simulink model "simulink_ompc_discrete"  (R2022b)
settings: Solver=ode8  StartTime=0.0  StopTime=time  FixedStep=Ts  RelTol=1e-3
values from neighbouring files (symbols this model uses):
  A_bar = [Ad, Z_unknown; zeros(n_disturbances, n_states), zeros(n_disturbances)]    [plik_generujDane.m]
  B_bar = [Bd; zeros(n_disturbances, size(Bd, 2))]    [plik_generujDane.m]
  Bd = Bd(:, 1:size(B, 2))    [plik_generujDane.m]
  C_bar = [C_measured, zeros(size(C_measured, 1), n_disturbances)]    [plik_generujDane.m]
  C_measured = [C_measured zeros(size(C_measured,1),1)]    [plik_generujDane.m]
  D = Dm    [generateBuilding.m]    (also in generateFloor.m; generateRoom.m = 0; heatPump.m = 0; mergePumpBuilding.m)
  K = P_pred * C' / (C * P_pred * C' + R)    [KalmanFilter.m]
  Kz = zeros(ny * na, nd * na)    [create_Kz_matrix.m]    (also in ompc_cost.m = [-K,eye(nu),zeros(nu,(nc-1)*nu)]; ompc_cost_tracking.m = [-K,eye(nu),zeros(nu,(nc-1)*nu),[K*Kxr+Kur zeros(nu,nya-nu)]; plik_generujDane.m = create_Kz_matrix(Ad, Cd, Zd, na))
  L = vecNeighbors(1,1)    [genRoomParams.m]    (also in generateParameters.m; generateRoom.m; model_expanded.m = 6; model_parameters.m)
  na = 72    [plik_generujDane.m]
  nc = 48    [plik_generujDane.m]
  npred = 72    [plik_generujDane.m]
  Qflow = table2array(roomEquipment(end,:))    [plik_generujDane.m]
  Sc = Spsi(nx+1:end,nx+1:end)    [ompc_cost.m]    (also in ompc_cost_tracking.m = Spsi(nx+1:nx+nuc,nx+1:nx+nuc))
  Scr = Spsi(nx+1:nx+nuc,nx+nuc+1:end)    [ompc_cost_tracking.m]
  Sxc = Spsi(1:nx,nx+1:end)    [ompc_cost.m]    (also in ompc_cost_tracking.m = Spsi(1:nx,nx+1:nx+nuc))
  time = 3600*24*7    (= 604800)    [plik_generujDane.m]
  trajDist = [d1Temp d2Temp d3Temp d4Temp d5Temp d6Temp d7Temp ... (first row only)    [plik_generujDane.m]
  trajPrice = [trajPrice trajPrice trajPrice trajPrice trajPrice trajPrice trajPrice]    [plik_generujDane.m]
  trajRef = [trajRef trajRef trajRef trajRef trajRef trajRef trajRef]    [plik_generujDane.m]
  Ts = 1200    [plik_generujDane.m]
  umax = [umax; P_MAX]    [plik_generujDane.m]
  umin = [umin; P_MIN]    [plik_generujDane.m]
  w_PumpCost = 1.5    [plik_generujDane.m]
  x0 = x0'    [initialStates.m]    (also in plik_generujDane.m = [x0;T_buf])
  xmax = [xmax [Ta_max xmax0 Twall_max Twall_max Tp_max T_return_max]]    [initialStates.m]    (also in plik_generujDane.m = [xmax; T_bufMAX])
  xmin = [xmin [Ta_min xmin0 Twall_min Twall_min Tp_min T_return_min]]    [initialStates.m]    (also in plik_generujDane.m = [xmin; T_bufMIN])
  ymax = [ymax; T_bufMAX]    [plik_generujDane.m]
  ymin = [ymin; T_bufMIN]    [plik_generujDane.m]
  Z = [Z zeros(nZ, nZmcol-3); Zm(:,1:2) zeros(nZm, nZcol-3) Zm(:,3:end)]    [generateBuilding.m]    (also in generateFloor.m = [Z zeros(nZ,1); Zm(:,1:2) zeros(nZm,nZcol-2) Zm(:,3)]; generateRoom.m = [0 0 0 0 0 0 1/Ca; heatPump.m = [area_buf*U -m_dot.*cw m_dot.*cw]/C_bufor; mergeFloorModels.m = Z0)
  Z_bar_known = [Z_known; zeros(n_disturbances, size(Z_known, 2))]    [plik_generujDane.m]
  Zd = Bd(:, size(B,2)+1:end)    [plik_generujDane.m]
  zoneWaterIndex = [zoneWaterIndex size(A,1)-1]    [plik_generujDane.m]
undefined symbols (not defined in the file or in its folder): Ad, Cd, priceCost
settings Model: Creator=artur  LastModifiedBy=artur

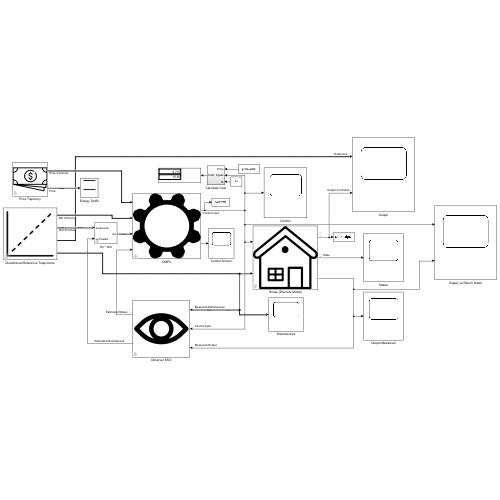
[thumbnail: Simulink's stored preview of the top-level diagram]
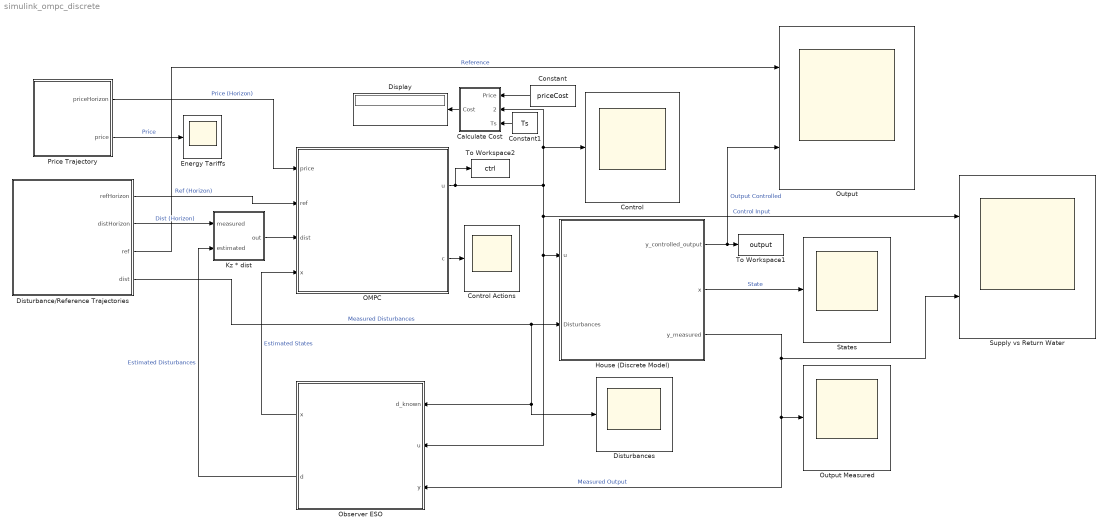
== system simulink_ompc_discrete ==
  Calculate Cost : Subsystem
  Constant : Constant  Value=priceCost
  Constant1 : Constant  Value=Ts
  Control : Scope
  Control Actions : Scope
  Display : Display
  Disturbance/Reference Trajectories : Subsystem  mask{time=time, Ts=Ts, na=na, refValues=trajRef, distValues=trajDist}
      mask prompts: time "Czas symulacji"; Ts "Okres próbkowania"; na "Horyzont trajektorii"; refValues "Trajektoria referencyjna"; distValues "Trajektoria zakłóceń"
      mask Display: image('C:\Users\artur\OneDrive\Dokumenty\MATLAB\Magisterka\model\images\plot-icon.svg'); % Use "Edit Image" on toolstrip to change.
  Disturbances : Scope
  Energy Tariffs : Scope
  House (Discrete Model) : Subsystem  mask{A=Ad, B=Bd, C=Cd, C_measured=C_measured, D=D, Z=Zd, x0=x0}
      mask prompts: A "Macierz A:"; B "Macierz B"; C "Macierz C sterowane"; C_measured "Macierz C mierzone"; D "Macierz D"; Z "Macierz zakłóceń Z"; x0 "War. początkowe"
      mask DialogControl ParameterGroupVar Prompt: Parametry modelu
      mask Display: image('C:\Users\artur\OneDrive\Dokumenty\MATLAB\Magisterka\model\images\house-icon.svg'); % Use "Edit Image" on toolstrip to change.
  Kz * dist : Subsystem  mask{Kz=Kz, na=na}
  OMPC : Subsystem  mask{A=Ad, B=Bd, C=Cd, nc=nc, npred=npred, na=na, w=w_PumpCost, Sxc=Sxc, Scr=Scr, Sc=Sc, K=K, umax=umax, umin=umin, ymax=ymax, ymin=ymin, xmax=xmax, xmin=xmin, M=zoneWaterIndex, Qflow=Qflow}
      mask prompts: A "Macierz A"; B "Macierz  B"; C "Macierz C"; nc "Liczba zmiennych decyzyjnych"; npred "Horyzont predykcji"; na "Horyzont trajektorii"; w "Waga kosztów cen energii"; Sxc "Macierz Sxc"; Scr "Macierz Scr"; Sc "Macierz Sc"; K "Macierz K"; M "Wektor indeksów stanów wody w strefie"; Qflow "PPrzepływy w pętlach grzewczych"
      mask DialogControl ParameterGroupVar Prompt: Parametry modelu
      mask DialogControl Container3 Prompt: Parametry regulatora
      mask DialogControl Container4 Prompt: Ograniczenia
      mask Display: image('C:\Users\artur\OneDrive\Dokumenty\MATLAB\Magisterka\model\images\cogwheel-icon.svg'); % Use "Edit Image" on toolstrip to change.
  Observer ESO : Subsystem  mask{A_bar=A_bar, B_bar=B_bar, C_bar=C_bar, A=Ad, L=L, Z_bar_known=Z_bar_known}
      mask DialogControl Observer Prompt: Parametry Obserwatora
      mask Display: image('C:\Users\artur\OneDrive\Dokumenty\MATLAB\Magisterka\model\images\eye-icon.svg'); % Use "Edit Image" on toolstrip to change.
  Output : Scope  NumInputPorts=2
  Output Measured : Scope
  Price Trajectory : Subsystem  mask{time=time, Ts=Ts, N=nc, refValues=trajPrice}
      mask prompts: time "Czas symulacji"; Ts "Okres próbkowania"; N "Horyzont"; refValues "Trajektoria zmian cen"
      mask Display: image('C:\Users\artur\OneDrive\Dokumenty\MATLAB\Magisterka\model\images\cash-icon.svg'); % Use "Edit Image" on toolstrip to change.
  States : Scope
  Supply vs Return Water : Scope  NumInputPorts=2
  To Workspace1 : ToWorkspace  VariableName=output  SampleTime=-1
      settings: Save2DSignal=2-D array (concatenate along first dimension)
  To Workspace2 : ToWorkspace  VariableName=ctrl  SampleTime=-1
      settings: Save2DSignal=2-D array (concatenate along first dimension)
  wires:
  OMPC/1(u) -> To Workspace2/1, Control/1, Calculate Cost/2(Inputs), Supply vs Return Water/1, House (Discrete Model)/1(u), Observer ESO/2(u)  "Control Input"
  House (Discrete Model)/2(x) -> States/1  "State"
  Disturbance/Reference Trajectories/3(ref) -> Output/1  "Reference"
  Disturbance/Reference Trajectories/1(refHorizon) -> OMPC/2(ref)  "Ref (Horizon)"
  House (Discrete Model)/3(y_measured) -> Supply vs Return Water/2, Output Measured/1, Observer ESO/3(y)  "Measured Output"
  Observer ESO/2(d) -> Kz * dist/2(estimated)  "Estimated Disturbances"
  House (Discrete Model)/1(y_controlled_output) -> Output/2, To Workspace1/1  "Output Controlled"
  Kz * dist/1(out) -> OMPC/3(dist)
  Disturbance/Reference Trajectories/2(distHorizon) -> Kz * dist/1(measured)  "Dist (Horizon)"
  OMPC/2(c) -> Control Actions/1
  Disturbance/Reference Trajectories/4(dist) -> Disturbances/1, Observer ESO/1(d_known), House (Discrete Model)/2(Disturbances)  "Measured Disturbances"
  Price Trajectory/1(priceHorizon) -> OMPC/1(price)  "Price (Horizon)"
  Price Trajectory/2(price) -> Energy Tariffs/1  "Price"
  Calculate Cost/1(Cost) -> Display/1
  Constant/1 -> Calculate Cost/1(Price)
  Constant1/1 -> Calculate Cost/3(Ts)
  Observer ESO/1(x) -> OMPC/4(x)  "Estimated States"

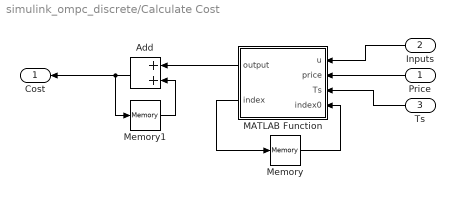
== system simulink_ompc_discrete/Calculate Cost ==
  Price : Inport
  Inputs : Inport  Port=2
  Ts : Inport  Port=3
  Add : Sum
  MATLAB Function : MATLAB Function  TreatAsAtomicUnit=on
  Memory : Memory  InitialCondition=1
  Memory1 : Memory  InitialCondition=[0 0]
  Cost : Outport
  wires:
  Inputs/1 -> MATLAB Function/1(u)
  Price/1 -> MATLAB Function/2(price)
  MATLAB Function/2(index) -> Memory/1
  Memory/1 -> MATLAB Function/4(index0)
  Memory1/1 -> Add/2
  Add/1 -> Cost/1, Memory1/1
  MATLAB Function/1(output) -> Add/1
  Ts/1 -> MATLAB Function/3(Ts)

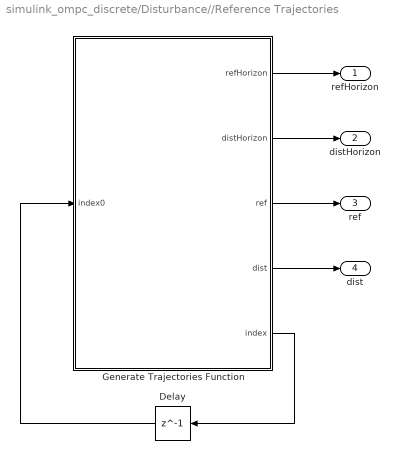
== system simulink_ompc_discrete/Disturbance//Reference Trajectories ==
  Delay : Delay  DelayLength=1  InitialCondition=1
  Generate Trajectories Function : MATLAB Function  TreatAsAtomicUnit=on
  refHorizon : Outport
  distHorizon : Outport  Port=2
  ref : Outport  Port=3
  dist : Outport  Port=4
  wires:
  Generate Trajectories Function/2(distHorizon) -> distHorizon/1
  Generate Trajectories Function/3(ref) -> ref/1
  Generate Trajectories Function/1(refHorizon) -> refHorizon/1
  Generate Trajectories Function/5(index) -> Delay/1
  Delay/1 -> Generate Trajectories Function/1(index0)
  Generate Trajectories Function/4(dist) -> dist/1

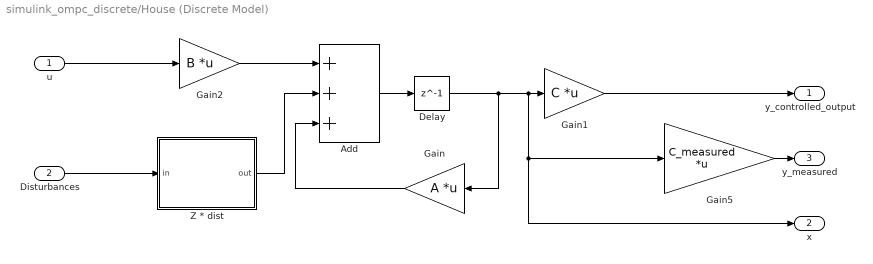
== system simulink_ompc_discrete/House (Discrete Model) ==
  u : Inport
  Disturbances : Inport  Port=2
  Add : Sum  Inputs=+++
  Delay : Delay  DelayLength=1  InitialCondition=x0
  Gain : Gain  Gain=A  Multiplication=Matrix(K*u) (u vector)
  Gain1 : Gain  Gain=C  Multiplication=Matrix(K*u) (u vector)
  Gain2 : Gain  Gain=B  Multiplication=Matrix(K*u) (u vector)
  Gain5 : Gain  Gain=C_measured  Multiplication=Matrix(K*u) (u vector)
  Z * dist : Subsystem  mask{Z=Z}
  y_controlled_output : Outport
  x : Outport  Port=2
  y_measured : Outport  Port=3
  wires:
  u/1 -> Gain2/1
  Delay/1 -> Gain5/1, x/1, Gain1/1, Gain/1
  Add/1 -> Delay/1
  Gain2/1 -> Add/1
  Gain1/1 -> y_controlled_output/1
  Gain/1 -> Add/3
  Disturbances/1 -> Z * dist/1(in)
  Z * dist/1(out) -> Add/2
  Gain5/1 -> y_measured/1

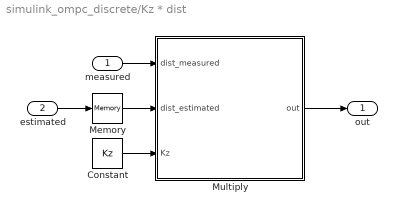
== system simulink_ompc_discrete/Kz * dist ==
  measured : Inport
  estimated : Inport  Port=2
  Constant : Constant  Value=Kz
  Memory : Memory  InitialCondition=zeros(size(Z,2)-6,1)
  Multiply : MATLAB Function  TreatAsAtomicUnit=on
  out : Outport
  wires:
  Multiply/1(out) -> out/1
  measured/1 -> Multiply/1(dist_measured)
  estimated/1 -> Memory/1
  Memory/1 -> Multiply/2(dist_estimated)
  Constant/1 -> Multiply/3(Kz)

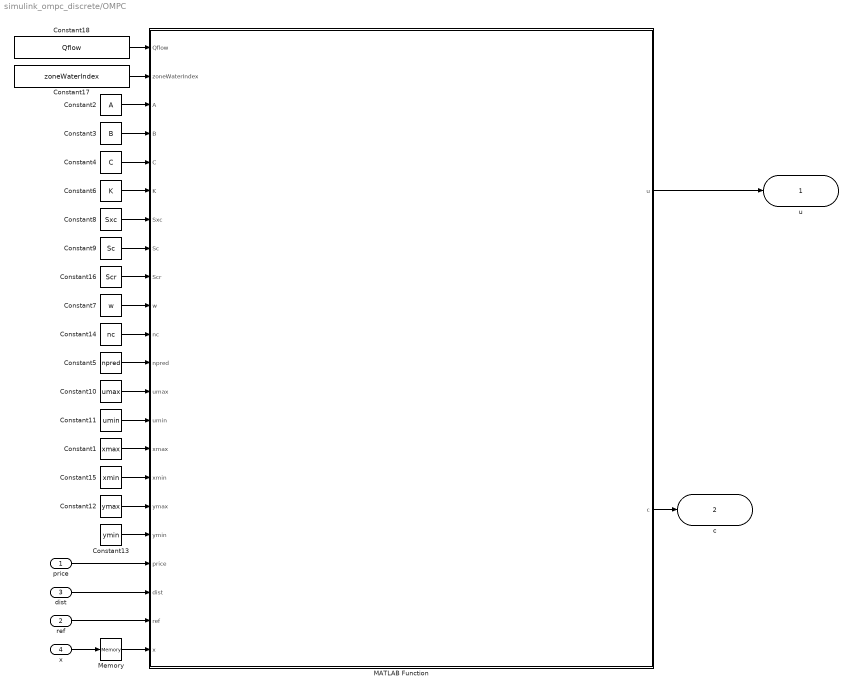
== system simulink_ompc_discrete/OMPC ==
  price : Inport
  ref : Inport  Port=2
  dist : Inport  Port=3
  x : Inport  Port=4
  Constant1 : Constant  Value=xmax  VectorParams1D=off
  Constant10 : Constant  Value=umax  VectorParams1D=off
  Constant11 : Constant  Value=umin  VectorParams1D=off
  Constant12 : Constant  Value=ymax
  Constant13 : Constant  Value=ymin
  Constant14 : Constant  Value=nc
  Constant15 : Constant  Value=xmin
  Constant16 : Constant  Value=Scr  VectorParams1D=off
  Constant17 : Constant  Value=zoneWaterIndex
  Constant18 : Constant  Value=Qflow
  Constant2 : Constant  Value=A
  Constant3 : Constant  Value=B  VectorParams1D=off
  Constant4 : Constant  Value=C  VectorParams1D=off
  Constant5 : Constant  Value=npred
  Constant6 : Constant  Value=K  VectorParams1D=off
  Constant7 : Constant  Value=w
  Constant8 : Constant  Value=Sxc  VectorParams1D=off
  Constant9 : Constant  Value=Sc  VectorParams1D=off
  MATLAB Function : MATLAB Function  TreatAsAtomicUnit=on
  Memory : Memory  InitialCondition=x0
  u : Outport
  c : Outport  Port=2
  wires:
  Constant6/1 -> MATLAB Function/6(K)
  Constant9/1 -> MATLAB Function/8(Sc)
  Constant8/1 -> MATLAB Function/7(Sxc)
  Constant2/1 -> MATLAB Function/3(A)
  Constant4/1 -> MATLAB Function/5(C)
  x/1 -> Memory/1
  Constant3/1 -> MATLAB Function/4(B)
  ref/1 -> MATLAB Function/21(ref)
  Constant10/1 -> MATLAB Function/13(umax)
  Constant11/1 -> MATLAB Function/14(umin)
  Constant12/1 -> MATLAB Function/17(ymax)
  Constant13/1 -> MATLAB Function/18(ymin)
  Memory/1 -> MATLAB Function/22(x)
  MATLAB Function/2(c) -> c/1
  Constant5/1 -> MATLAB Function/12(npred)
  Constant14/1 -> MATLAB Function/11(nc)
  dist/1 -> MATLAB Function/20(dist)
  Constant15/1 -> MATLAB Function/16(xmin)
  Constant1/1 -> MATLAB Function/15(xmax)
  Constant16/1 -> MATLAB Function/9(Scr)
  price/1 -> MATLAB Function/19(price)
  Constant7/1 -> MATLAB Function/10(w)
  Constant17/1 -> MATLAB Function/2(zoneWaterIndex)
  Constant18/1 -> MATLAB Function/1(Qflow)
  MATLAB Function/1(u) -> u/1

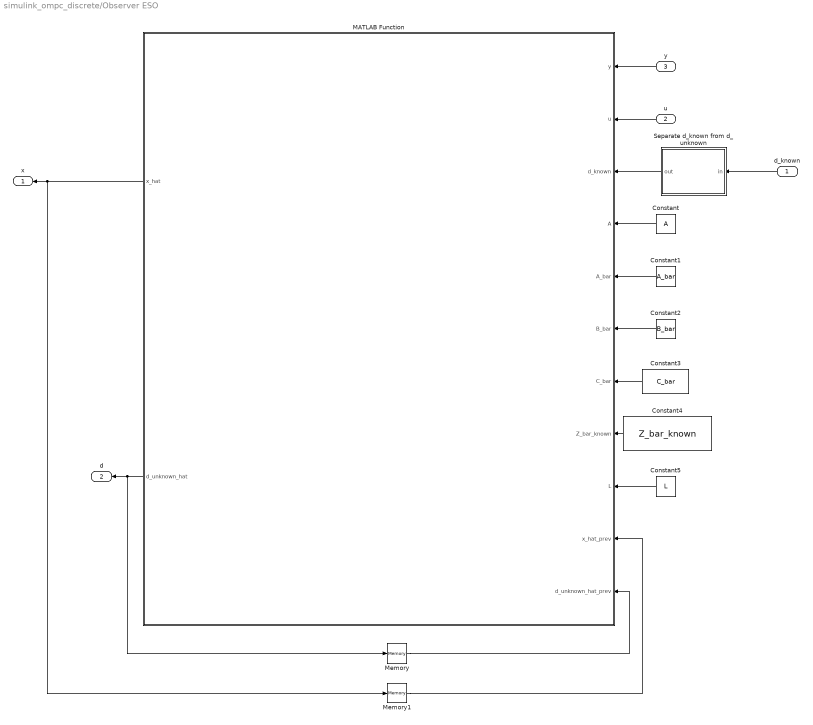
== system simulink_ompc_discrete/Observer ESO ==
  d_known : Inport
  u : Inport  Port=2
  y : Inport  Port=3
  Constant : Constant  Value=A
  Constant1 : Constant  Value=A_bar
  Constant2 : Constant  Value=B_bar
  Constant3 : Constant  Value=C_bar
  Constant4 : Constant  Value=Z_bar_known
  Constant5 : Constant  Value=L
  MATLAB Function : MATLAB Function  TreatAsAtomicUnit=on
  Memory : Memory  InitialCondition=zeros(size(Z,2) - size(Z_bar_known,2),1)
  Memory1 : Memory  InitialCondition=x0
  Separate d_known from d_unknown : MATLAB Function  TreatAsAtomicUnit=on
  x : Outport
  d : Outport  Port=2
  wires:
  MATLAB Function/2(d_unknown_hat) -> Memory/1, d/1
  Memory/1 -> MATLAB Function/11(d_unknown_hat_prev)
  Memory1/1 -> MATLAB Function/10(x_hat_prev)
  MATLAB Function/1(x_hat) -> Memory1/1, x/1
  y/1 -> MATLAB Function/1(y)
  u/1 -> MATLAB Function/2(u)
  Constant/1 -> MATLAB Function/4(A)
  Constant1/1 -> MATLAB Function/5(A_bar)
  Constant2/1 -> MATLAB Function/6(B_bar)
  Constant3/1 -> MATLAB Function/7(C_bar)
  Constant4/1 -> MATLAB Function/8(Z_bar_known)
  Constant5/1 -> MATLAB Function/9(L)
  d_known/1 -> Separate d_known from d_unknown/1(in)
  Separate d_known from d_unknown/1(out) -> MATLAB Function/3(d_known)

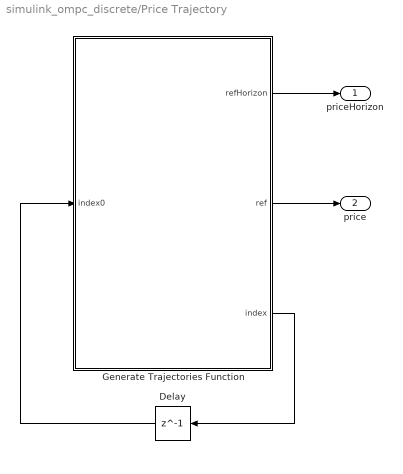
== system simulink_ompc_discrete/Price Trajectory ==
  Delay : Delay  DelayLength=1  InitialCondition=1
  Generate Trajectories Function : MATLAB Function  TreatAsAtomicUnit=on
  priceHorizon : Outport
  price : Outport  Port=2
  wires:
  Generate Trajectories Function/2(ref) -> price/1
  Generate Trajectories Function/1(refHorizon) -> priceHorizon/1
  Generate Trajectories Function/3(index) -> Delay/1
  Delay/1 -> Generate Trajectories Function/1(index0)

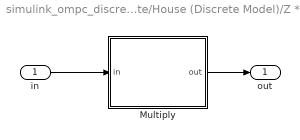
== system simulink_ompc_discrete/House (Discrete Model)/Z * dist ==
  in : Inport
  Multiply : MATLAB Function  TreatAsAtomicUnit=on
  out : Outport
  wires:
  Multiply/1(out) -> out/1
  in/1 -> Multiply/1(in)

== matlab function simulink_ompc_discrete/Observer ESO/MATLAB Function ==
  data: y input; u input; x_hat output; d_unknown_hat output; d_known input; A input; A_bar input; B_bar input; C_bar input; Z_bar_known input; L input; x_hat_prev input; d_unknown_hat_prev input
function [x_hat, d_unknown_hat] = observerESO(y, u, d_known, A, A_bar, B_bar, C_bar, Z_bar_known, L, x_hat_prev, d_unknown_hat_prev)

nx = size(A, 1);

% Rozszerzone stany
x_bar_hat = [x_hat_prev; d_unknown_hat_prev];
y_hat = C_bar * x_bar_hat;

% Aktualizacja estymacji
x_bar_hat = A_bar * x_bar_hat + B_bar * u + Z_bar_known * d_known + L * (y - y_hat);

x_hat = x_bar_hat(1:nx); % Estymowane stany
d_unknown_hat = x_bar_hat(nx+1:end); % Estymowane nieznane zakłócenia
end

== matlab function simulink_ompc_discrete/Observer ESO/Separate d_known from d_unknown ==
  data: in input; out output
function out = fcn(in)

out = in(1:6,:);

== matlab function simulink_ompc_discrete/House (Discrete Model)/Z * dist/Multiply ==
  data: in input; out output; Z parameter
function out = fcn(in, Z)
out = Z*in;

== matlab function simulink_ompc_discrete/Price Trajectory/Generate Trajectories Function ==
  data: refHorizon output size=na*ny; ref output size=ny; time parameter; Ts parameter; N parameter; refValues parameter; index output; index0 input
function [refHorizon,ref,index] = fcn(time, Ts, N, refValues, index0)

flag = 1;
[~, refHorizon, ref] = generateTrajectory(refValues,flag,time,Ts,N,index0);

index = index0 + 1;

== matlab function simulink_ompc_discrete/Calculate Cost/MATLAB Function ==
  data: u input; output output; price input; Ts input; index0 input; index output
function [output, index] = fcn(u, price, Ts, index0)

% u [W]
% price [kWh]

%przekonwertuj na kWh
t_base = Ts/3600;

cost = u(end,end)/1000*t_base * price(index0);
power = u(end,end)/1000*t_base;
output = [cost power];
index = index0 + 1;

== matlab function simulink_ompc_discrete/Disturbance//Reference Trajectories/Generate Trajectories Function ==
  data: refHorizon output size=na*ny; distHorizon output size=na*nz; ref output size=ny; dist output size=nz; time parameter; Ts parameter; na parameter; refValues parameter; distValues parameter; index output; index0 input
function [refHorizon,distHorizon,ref,dist,index] = fcn(time, Ts, na, refValues, distValues, index0)

mode = 1;
[~, refHorizon, ref] = generateTrajectory(refValues,mode,time,Ts,na,index0);

N = size(refValues,1);

for i = 1:N-1
    for j = 1:na-1
        if refHorizon(i + (j-1)*N) > refHorizon(i+j*N)
            refHorizon(i+j*N) = refHorizon(i + (j-1)*N);
        end
    end
end

mode = 2;
[~, distHorizon, dist] = generateTrajectory(distValues,mode,time,Ts,na,index0);

index = index0 + 1;

== matlab function simulink_ompc_discrete/Kz * dist/Multiply ==
  data: dist_measured input; dist_estimated input; out output size=ny*na; Kz input
function out = fcn(dist_measured,dist_estimated, Kz)

%--------------------------------------------------------------------------
%Stwórz wektor sygnałów zakłócających z danych pomiarowych oraz estymacji
len_measured = length(dist_measured);
len_estimated = length(dist_estimated);
len_repeating = 6 + len_estimated; %6 wynika z liczby zakłóceń mierzalnych
N = len_measured / len_repeating;
disturbance_vector = zeros(size(dist_measured));
idx = 1;
for i = 1:N
    start_idx = (i-1) * len_repeating + 1;
    disturbance_vector(idx:idx+2) = dist_measured(start_idx:start_idx+2);
    idx = idx + 6;
    disturbance_vector(idx:idx+len_estimated-1) = dist_estimated;
    idx = idx + len_estimated;
end

out = Kz*disturbance_vector;

== matlab function simulink_ompc_discrete/OMPC/MATLAB Function ==
  data: Qflow input; zoneWaterIndex input; A input; B input; C input; K input; Sxc input; Sc input; Scr input; w input; nc input; npred input; umax input; umin input; xmax input; xmin input; ymax input; ymin input; price input; dist input; ref input; x input; u output; c output
function [u,c] = fcn(Qflow,zoneWaterIndex,A,B,C,K,Sxc,Sc,Scr,w,nc,npred,umax,umin,xmax,xmin,ymax,ymin,price,dist,ref,x)

for i = 1:size(umin,1)-1
    umin(i) = x(zoneWaterIndex(i));
end

[u,ctrl] = ompc_law(A,B,C,K,Sxc,Sc,Scr,Qflow,zoneWaterIndex,umax,umin,xmax,xmin,ymax,ymin,w,nc,npred,price,ref,dist,x);
c = ctrl(1:size(B,2),:);
